simulink library "MATH_library"  (R2018b)
settings: Solver=VariableStepAuto  StartTime=0.0  StopTime=10.0  RelTol=1e-3
undefined symbols (not defined in the file): Newton, Raphson
libraries: $bdroot x48, sharedutil x4
(part 1 of 2)
settings Model: Creator=Andrea  LastModifiedBy=michele

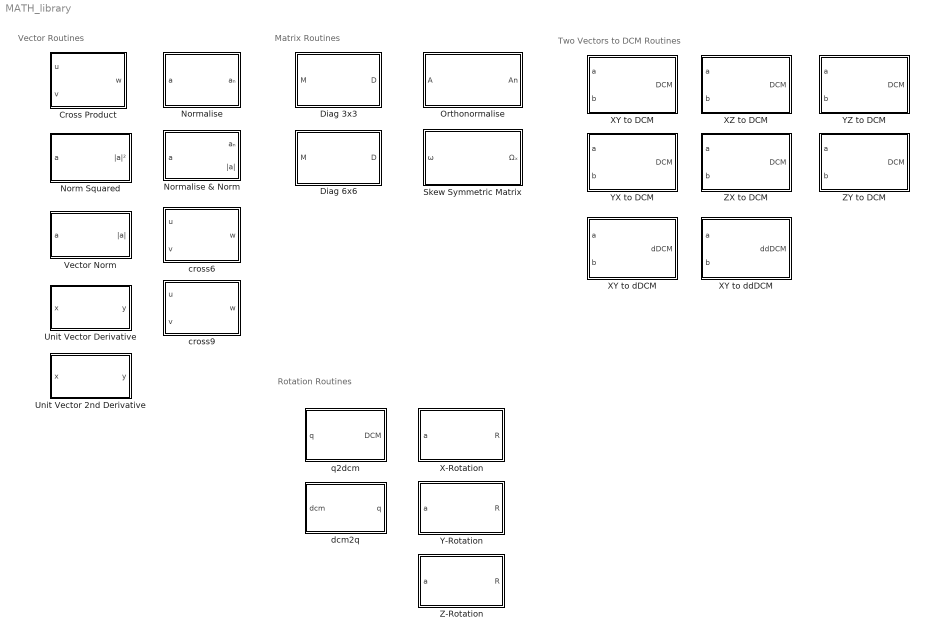
== system MATH_library ==
  note: Rotation Routines
  note: Matrix Routines
  note: Vector Routines
  note: Two Vectors to DCM Routines
  Cross Product : Subsystem  mask(Cross Product){}
      mask help: This block computes the cross product between two 3x1 input vectors u and v. The output vector w is such that w = u x v
  Diag 3x3 : Subsystem  mask(Diagonal - 3x3){}
      mask help: Extract the diagonal of a 3x3 matrix.
  Diag 6x6 : Subsystem  mask(Diagonal - 6x6){}
      mask help: Extract the diagonal of a 6x6 matrix.
  Norm Squared : Subsystem  mask(Norm Squared){}
      mask help: Compute the square of the norm of the input vector.
  Normalise : Subsystem  mask(Normalise){}
      mask help: Normalise the input vector.
  Normalise & Norm : Subsystem  mask(Normalise){}
      mask help: Normalise the input vector and also return its norm.
  Orthonormalise : Subsystem  mask(Matrix Orthonormalisation){}
      mask help: This block performs the Gram-Schmidt orthonormalisation process on the input matrix A. However, note that this block does not check whether the columns of A span a three-dimensional space.
  Skew Symmetric Matrix : Subsystem  mask(Skew Symmetric Matrix){}
      mask help: This block generates a skew-symmetric matrix W from the given input vector w. The output matrix is defined such that the cross product w x b can be written as W * b
  Unit Vector 2nd Derivative : Subsystem  mask(Unit vector derivative){}
      mask help: Compute the derivative of a unit vector.
  Unit Vector Derivative : Subsystem  mask(Unit vector derivative){}
      mask help: Compute the derivative of a unit vector.
  Vector Norm : Subsystem  mask(Vector Norm){}
      mask help: Compute the norm of the input vector.
  X-Rotation : Subsystem  mask(X - Rotation){}
      mask help: Compute the matrix for a PASSIVE rotation around the X-axis for a given angle [rad].
  XY to DCM : Subsystem  mask(XY to DCM){}
      mask help:
      | This block computes a DCM from a 3D right-handed orthogonal vector basis obtained from the input vector a and b.
      |
      | INPUTS:
      |   - Primary vector that will be aligned with the X-axis
      |   - Secondary vector. The component of this vector that is orthogonal to the primary vector will be aligned to the Y-axis.
      |
      | OUTPUTS:
      |  -  3x3 Rotation matrix from the axes in which a and b are defined to the new ones.
  XY to dDCM : Subsystem  mask(XY to dDCM){}
      mask help:
      | This block computes the derivative of a DCM from a 3D right-handed orthogonal vector basis obtained from the input vector a and b. These input vectors must be of 6-elements, with the last 3 the derivatives of the first three.
      |
      | INPUTS:
      |   - Primary vector that will be aligned with the X-axis.
      |   - Secondary vector. The component of this vector that is orthogonal to the primary vector will be aligned to the Y-axis.
      |
      | OUTPUTS:
      |  -  3x3 Rotation matrix from the axes in which a and b are defined to the new ones.
  XY to ddDCM : Subsystem  mask(XY to dDCM){}
      mask help:
      | This block computes the derivative of a DCM from a 3D right-handed orthogonal vector basis obtained from the input vector a and b. These input vectors must be of 6-elements, with the last 3 the derivatives of the first three.
      |
      | INPUTS:
      |   - Primary vector that will be aligned with the X-axis.
      |   - Secondary vector. The component of this vector that is orthogonal to the primary vector will be aligned to the Y-axis.
      |
      | OUTPUTS:
      |  -  3x3 Rotation matrix from the axes in which a and b are defined to the new ones.
  XZ to DCM : Subsystem  mask(XZ to DCM){}
      mask help:
      | This block computes a DCM from a 3D right-handed orthogonal vector basis obtained from the input vector a and b.
      |
      | INPUTS:
      |   - Primary vector that will be aligned with the X-axis
      |   - Secondary vector. The component of this vector that is orthogonal to the primary vector will be aligned to the Z-axis.
      |
      | OUTPUTS:
      |   -  3x3 Rotation matrix from the axes in which a and b are defined to the new ones.
  Y-Rotation : Subsystem  mask(Y - Rotation){}
      mask help: Compute the matrix for a PASSIVE rotation around the Y-axis for a given angle [rad].
  YX to DCM : Subsystem  mask(YX to DCM){}
      mask help:
      | This block computes a DCM from a 3D right-handed orthogonal vector basis obtained from the input vector a and b.
      |
      | INPUTS:
      |   - Primary vector that will be aligned with the Y-axis
      |   - Secondary vector. The component of this vector that is orthogonal to the primary vector will be aligned to the X-axis.
      |
      | OUTPUTS:
      |   -  3x3 Rotation matrix from the axes in which a and b are defined to the new ones.
  YZ to DCM : Subsystem  mask(YZ to DCM){}
      mask help:
      | This block computes a DCM from a 3D right-handed orthogonal vector basis obtained from the input vector a and b.
      |
      | INPUTS:
      |   - Primary vector that will be aligned with the Y-axis
      |   - Secondary vector. The component of this vector that is orthogonal to the primary vector will be aligned to the Z-axis.
      |
      | OUTPUTS:
      |   -  3x3 Rotation matrix from the axes in which a and b are defined to the new ones.
  Z-Rotation : Subsystem  mask(Z - Rotation){}
      mask help: Compute the matrix for a PASSIVE rotation around the Z-axis for a given angle [rad].
  ZX to DCM : Subsystem  mask(ZX to DCM){}
      mask help:
      | This block computes a DCM from a 3D right-handed orthogonal vector basis obtained from the input vector a and b.
      |
      | INPUTS:
      |   - Primary vector that will be aligned with the Z-axis
      |   - Secondary vector. The component of this vector that is orthogonal to the primary vector will be aligned to the X-axis.
      |
      | OUTPUTS:
      |   -  3x3 Rotation matrix from the axes in which a and b are defined to the new ones.
  ZY to DCM : Subsystem  mask(ZY to DCM){}
      mask help:
      | This block computes a DCM from a 3D right-handed orthogonal vector basis obtained from the input vector a and b.
      |
      | INPUTS:
      |   - Primary vector that will be aligned with the Z-axis
      |   - Secondary vector. The component of this vector that is orthogonal to the primary vector will be aligned to the Y-axis.
      |
      | OUTPUTS:
      |   -  3x3 Rotation matrix from the axes in which a and b are defined to the new ones.
  cross6 : Subsystem  mask(Cross 6){}
      mask help: Compute the cross product between two vectors and its time derivative. Each input vector must be of 6 elements, with the last 3 that represent the derivative of the first.
  cross9 : Subsystem  mask(Cross 6){}
      mask help: Compute the cross product between two vectors and its time derivative. Each input vector must be of 6 elements, with the last 3 that represent the derivative of the first.
  dcm2q : Subsystem  mask(DCM to Quaternion){}
      mask help: Convert a Direction Cosine Matrix (DCM) into a quaternion (in scalar-last format).
  q2dcm : Subsystem  mask(Quaternion to DCM){}
      mask help: Convert a quaternion (in scalar-last format) into a Direction Cosine Matrix (DCM)

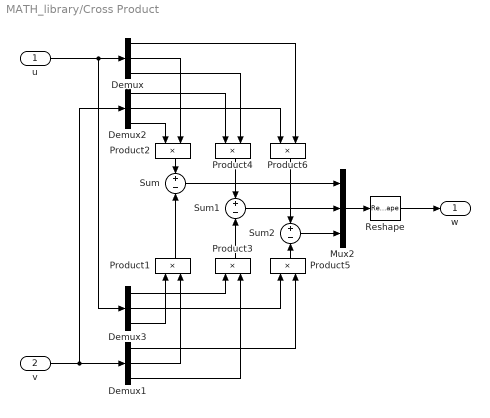
== system MATH_library/Cross Product ==
  u : Inport
  v : Inport  Port=2
  Demux{,1..3} (4 alike) : Demux  Outputs=3
  Mux2 : Mux  Inputs=3
  Product{1..6} (6 alike) : Product  SaturateOnIntegerOverflow=on  RndMeth=Zero  InputSameDT=on  OutDataTypeStr=Inherit: Same as first input
  Reshape : Reshape  OutputDimensionality=Column vector (2-D)
  Sum : Sum  Inputs=+-  SaturateOnIntegerOverflow=on  InputSameDT=on  OutDataTypeStr=Inherit: Same as first input
  Sum1 : Sum  Inputs=+-  SaturateOnIntegerOverflow=on  InputSameDT=on  OutDataTypeStr=Inherit: Same as first input
  Sum2 : Sum  Inputs=+-  SaturateOnIntegerOverflow=on  InputSameDT=on  OutDataTypeStr=Inherit: Same as first input
  w : Outport
  wires:
  Product6/1 -> Sum2/1
  Demux/2 -> Product2/2
  Demux2/1 -> Product4/1
  Product1/1 -> Sum/2
  Product4/1 -> Sum1/1
  Sum2/1 -> Mux2/3
  Sum1/1 -> Mux2/2
  Demux3/3 -> Product1/1
  u/1 -> Demux3/1, Demux/1
  Demux/3 -> Product4/2
  Product3/1 -> Sum1/2
  Mux2/1 -> Reshape/1
  Demux/1 -> Product6/2
  Demux1/2 -> Product1/2
  Product5/1 -> Sum2/2
  Sum/1 -> Mux2/1
  Demux1/1 -> Product5/2
  Product2/1 -> Sum/1
  Reshape/1 -> w/1
  v/1 -> Demux1/1, Demux2/1
  Demux2/2 -> Product6/1
  Demux1/3 -> Product3/2
  Demux3/2 -> Product5/1
  Demux3/1 -> Product3/1
  Demux2/3 -> Product2/1

== system MATH_library/Diag 3x3 ==
  M : Inport  OutDataTypeStr=single  PortDimensions=[3,3]
  Reshape : Reshape
  Selector : Selector  InputPortWidth=9  IndexOptions=Index vector (dialog)  Indices=[1 5 9]  OutputSizes=1
  D : Outport  OutDataTypeStr=single  PortDimensions=3
  wires:
  M/1 -> Reshape/1
  Reshape/1 -> Selector/1
  Selector/1 -> D/1

== system MATH_library/Diag 6x6 ==
  M : Inport  PortDimensions=[6,6]
  Reshape : Reshape
  Selector : Selector  InputPortWidth=36  IndexOptions=Index vector (dialog)  Indices=[1 8 15 22 29 36]  OutputSizes=1
  D : Outport  PortDimensions=6
  wires:
  M/1 -> Reshape/1
  Reshape/1 -> Selector/1
  Selector/1 -> D/1

== system MATH_library/Norm Squared ==
  a : Inport
  Dot Product : DotProduct  InputSameDT=on  OutDataTypeStr=Inherit: Inherit via internal rule
  |a|² : Outport
  wires:
  a/1 -> Dot Product/2, Dot Product/1
  Dot Product/1 -> |a|²/1

== system MATH_library/Normalise ==
  a : Inport
  Divide : Product  Inputs=*/
  Vector Norm : $bdroot/Vector Norm
  aₙ : Outport
  wires:
  a/1 -> Vector Norm/1, Divide/1
  Divide/1 -> aₙ/1
  Vector Norm/1 -> Divide/2

== system MATH_library/Normalise & Norm ==
  a : Inport
  Divide : Product  Inputs=*/
  Vector Norm : $bdroot/Vector Norm
  aₙ : Outport
  |a| : Outport  Port=2
  wires:
  a/1 -> Vector Norm/1, Divide/1
  Divide/1 -> aₙ/1
  Vector Norm/1 -> |a|/1, Divide/2

== system MATH_library/Orthonormalise ==
  A : Inport
  Demux : Demux  Outputs=3
  Normalise : $bdroot/Normalise
  Reshape : Reshape  OutputDimensionality=Column vector (2-D)
  Subsystem : Subsystem
  Subsystem1 : Subsystem
  Vector Concatenate : Concatenate  NumInputs=3  Mode=Multidimensional array  ConcatenateDimension=2
  An : Outport
  wires:
  A/1 -> Reshape/1
  Reshape/1 -> Demux/1
  Demux/1 -> Normalise/1  "e1"
  Normalise/1 -> Subsystem1/1(en1), Subsystem/1(en1), Vector Concatenate/1
  Demux/2 -> Subsystem/2(e2)  "e2"
  Demux/3 -> Subsystem1/2(e3)  "e3"
  Subsystem1/1(en3) -> Vector Concatenate/3
  Subsystem/1(en2) -> Subsystem1/3(en2), Vector Concatenate/2
  Vector Concatenate/1 -> An/1

== system MATH_library/Skew Symmetric Matrix ==
  ω : Inport
  Constant : Constant  Value=0
  Demux : Demux  Outputs=3
  Gain : Gain  Gain=-1
  Gain1 : Gain  Gain=-1
  Gain2 : Gain  Gain=-1
  Reshape (9) to [3x3] column-major : Reshape  OutputDimensionality=Customize  OutputDimensions=[3,3]
  Vector Concatenate : Concatenate  NumInputs=9
  Ωₓ : Outport
  wires:
  Constant/1 -> Vector Concatenate/9, Vector Concatenate/5, Vector Concatenate/1
  Demux/1 -> Vector Concatenate/6, Gain/1
  Reshape (9) to [3x3] column-major/1 -> Ωₓ/1
  Demux/3 -> Gain2/1, Vector Concatenate/2
  Demux/2 -> Vector Concatenate/7, Gain1/1
  ω/1 -> Demux/1
  Vector Concatenate/1 -> Reshape (9) to [3x3] column-major/1
  Gain1/1 -> Vector Concatenate/3
  Gain2/1 -> Vector Concatenate/4
  Gain/1 -> Vector Concatenate/8

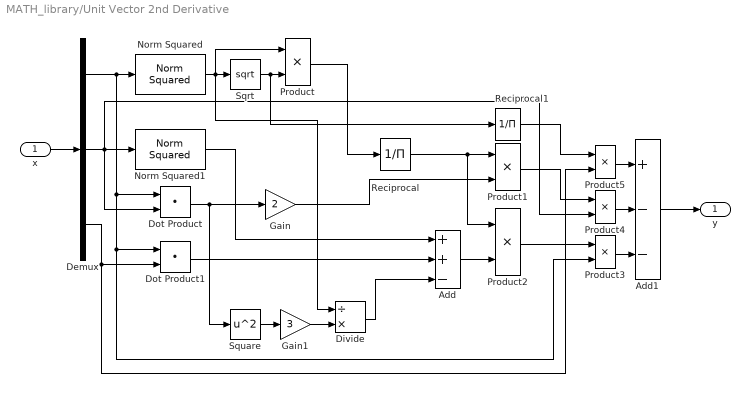
== system MATH_library/Unit Vector 2nd Derivative ==
  x : Inport
  Add : Sum  Inputs=++-
  Add1 : Sum  Inputs=+--
  Demux : Demux  Outputs=3
  Divide : Product  Inputs=/*
  Dot Product : DotProduct  InputSameDT=on  OutDataTypeStr=Inherit: Inherit via internal rule
  Dot Product1 : DotProduct  InputSameDT=on  OutDataTypeStr=Inherit: Inherit via internal rule
  Gain : Gain  Gain=2
  Gain1 : Gain  Gain=3
  Norm Squared : $bdroot/Norm Squared
  Norm Squared1 : $bdroot/Norm Squared
  Product{,1..5} (6 alike) : Product
  Reciprocal : Product  Inputs=/
  Reciprocal1 : Product  Inputs=/
  Sqrt : Sqrt  SaturateOnIntegerOverflow=on
  Square : Math  Operator=square  SaturateOnIntegerOverflow=on
  y : Outport
  wires:
  Add1/1 -> y/1
  x/1 -> Demux/1
  Demux/1 -> Norm Squared/1, Product3/2, Dot Product1/1, Dot Product/1
  Norm Squared/1 -> Divide/1, Product/1, Sqrt/1
  Sqrt/1 -> Reciprocal1/1, Product/2
  Demux/2 -> Product4/2, Dot Product/2, Norm Squared1/1
  Demux/3 -> Product5/2, Dot Product1/2
  Dot Product/1 -> Square/1, Gain/1
  Gain/1 -> Product1/2
  Reciprocal/1 -> Product2/1, Product1/1
  Product/1 -> Reciprocal/1
  Norm Squared1/1 -> Add/1
  Dot Product1/1 -> Add/2
  Square/1 -> Gain1/1
  Gain1/1 -> Divide/2
  Divide/1 -> Add/3
  Add/1 -> Product2/2
  Product2/1 -> Product3/1
  Product3/1 -> Add1/3
  Product4/1 -> Add1/2
  Product1/1 -> Product4/1
  Product5/1 -> Add1/1
  Reciprocal1/1 -> Product5/1

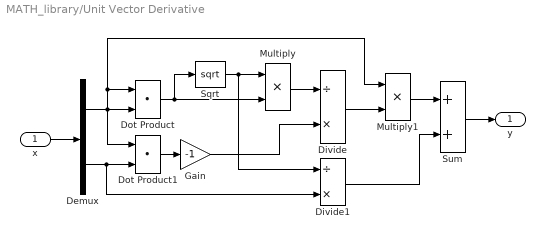
== system MATH_library/Unit Vector Derivative ==
  x : Inport
  Demux : Demux  Outputs=2
  Divide : Product  Inputs=/*
  Divide1 : Product  Inputs=/*
  Dot Product : DotProduct  InputSameDT=on  OutDataTypeStr=Inherit: Inherit via internal rule
  Dot Product1 : DotProduct  InputSameDT=on  OutDataTypeStr=Inherit: Inherit via internal rule
  Gain : Gain  Gain=-1
  Multiply : Product
  Multiply1 : Product
  Sqrt : Sqrt  SaturateOnIntegerOverflow=on
  Sum : Sum
  y : Outport
  wires:
  Divide/1 -> Multiply1/2
  Divide1/1 -> Sum/2
  Sum/1 -> y/1
  Multiply1/1 -> Sum/1
  Multiply/1 -> Divide/1
  Gain/1 -> Divide/2
  Demux/2 -> Divide1/2, Dot Product1/2
  Dot Product1/1 -> Gain/1
  Demux/1 -> Dot Product1/1, Multiply1/1, Dot Product/1, Dot Product/2
  Sqrt/1 -> Multiply/1, Divide1/1
  Dot Product/1 -> Multiply/2, Sqrt/1
  x/1 -> Demux/1

== system MATH_library/Vector Norm ==
  a : Inport
  Norm Squared : $bdroot/Norm Squared
  Sqrt : Sqrt  SaturateOnIntegerOverflow=on
  |a| : Outport
  wires:
  Sqrt/1 -> |a|/1
  Norm Squared/1 -> Sqrt/1
  a/1 -> Norm Squared/1

== system MATH_library/X-Rotation ==
  a : Inport
  Constant1 : Constant  Value=0
  Constant2 : Constant
  Constant3 : Constant  Value=0
  Constant4 : Constant
  Constant5 : Constant  Value=0
  Create 3x3 Matrix : sharedutil/Create 3x3 Matrix  aMode=aMode
  Gain : Gain  Gain=-1
  SinCos : Trigonometry  Operator=sincos
  R : Outport
  wires:
  a/1 -> SinCos/1
  Create 3x3 Matrix/1 -> R/1
  SinCos/2 -> Create 3x3 Matrix/9, Create 3x3 Matrix/5
  SinCos/1 -> Create 3x3 Matrix/6, Gain/1
  Constant3/1 -> Create 3x3 Matrix/2
  Constant4/1 -> Create 3x3 Matrix/1
  Constant5/1 -> Create 3x3 Matrix/3
  Constant2/1 -> Create 3x3 Matrix/7
  Constant1/1 -> Create 3x3 Matrix/4
  Gain/1 -> Create 3x3 Matrix/8

== system MATH_library/XY to DCM ==
  a : Inport
  b : Inport  Port=2
  " Matrix" : Concatenate  NumInputs=3  Mode=Multidimensional array  ConcatenateDimension=2
  Cross Product : $bdroot/Cross Product
  Cross Product1 : $bdroot/Cross Product
  Normalise : $bdroot/Normalise
  Normalise1 : $bdroot/Normalise
  Normalise2 : $bdroot/Normalise
  Transpose : Math  Operator=transpose  SaturateOnIntegerOverflow=on
  DCM : Outport
  wires:
  Normalise/1 -> " Matrix"/3  "w_n"
  Cross Product/1 -> Normalise/1, Cross Product1/1
  " Matrix"/1 -> Transpose/1
  Normalise2/1 -> " Matrix"/1  "u_n"
  Normalise1/1 -> " Matrix"/2  "v_n"
  b/1 -> Cross Product/2
  a/1 -> Normalise2/1, Cross Product/1, Cross Product1/2
  Cross Product1/1 -> Normalise1/1
  Transpose/1 -> DCM/1

== system MATH_library/XY to dDCM ==
  a : Inport
  b : Inport  Port=2
  " Matrix" : Concatenate  NumInputs=3  Mode=Multidimensional array  ConcatenateDimension=2
  Transpose : Math  Operator=transpose  SaturateOnIntegerOverflow=on
  Unit Vector Derivative : $bdroot/Unit Vector Derivative
  Unit Vector Derivative1 : $bdroot/Unit Vector Derivative
  Unit Vector Derivative2 : $bdroot/Unit Vector Derivative
  cross1 : $bdroot/cross6
  cross2 : $bdroot/cross6
  dDCM : Outport
  wires:
  Transpose/1 -> dDCM/1
  " Matrix"/1 -> Transpose/1
  cross2/1 -> Unit Vector Derivative1/1
  Unit Vector Derivative/1 -> " Matrix"/3
  cross1/1 -> Unit Vector Derivative/1, cross2/1
  b/1 -> cross1/2, cross2/2
  a/1 -> Unit Vector Derivative2/1, cross1/1
  Unit Vector Derivative2/1 -> " Matrix"/1
  Unit Vector Derivative1/1 -> " Matrix"/2

== system MATH_library/XY to ddDCM ==
  a : Inport
  b : Inport  Port=2
  " Matrix" : Concatenate  NumInputs=3  Mode=Multidimensional array  ConcatenateDimension=2
  Transpose : Math  Operator=transpose  SaturateOnIntegerOverflow=on
  Unit Vector 2nd Derivative : $bdroot/Unit Vector 2nd Derivative
  Unit Vector 2nd Derivative1 : $bdroot/Unit Vector 2nd Derivative
  Unit Vector 2nd Derivative2 : $bdroot/Unit Vector 2nd Derivative
  cross1 : $bdroot/cross9
  cross9 : $bdroot/cross9
  ddDCM : Outport
  wires:
  Transpose/1 -> ddDCM/1
  " Matrix"/1 -> Transpose/1
  cross1/1 -> Unit Vector 2nd Derivative1/1
  Unit Vector 2nd Derivative2/1 -> " Matrix"/3
  cross9/1 -> Unit Vector 2nd Derivative2/1, cross1/1
  b/1 -> cross1/2, cross9/2
  a/1 -> Unit Vector 2nd Derivative/1, cross9/1
  Unit Vector 2nd Derivative/1 -> " Matrix"/1
  Unit Vector 2nd Derivative1/1 -> " Matrix"/2

== system MATH_library/XZ to DCM ==
  a : Inport
  b : Inport  Port=2
  " Matrix" : Concatenate  NumInputs=3  Mode=Multidimensional array  ConcatenateDimension=2
  Cross Product1 : $bdroot/Cross Product
  Cross Product2 : $bdroot/Cross Product
  Normalise1 : $bdroot/Normalise
  Normalise2 : $bdroot/Normalise
  Normalise3 : $bdroot/Normalise
  Transpose : Math  Operator=transpose  SaturateOnIntegerOverflow=on
  DCM : Outport
  wires:
  Normalise1/1 -> " Matrix"/3  "w_n"
  " Matrix"/1 -> Transpose/1
  Normalise3/1 -> " Matrix"/1  "u_n"
  Normalise2/1 -> " Matrix"/2  "v_n"
  a/1 -> Normalise3/1, Cross Product2/2, Cross Product1/1
  Cross Product2/1 -> Cross Product1/2, Normalise2/1
  b/1 -> Cross Product2/1
  Cross Product1/1 -> Normalise1/1
  Transpose/1 -> DCM/1

== system MATH_library/Y-Rotation ==
  a : Inport
  Constant1 : Constant  Value=0
  Constant2 : Constant
  Constant3 : Constant  Value=0
  Constant4 : Constant
  Constant5 : Constant  Value=0
  Create 3x3 Matrix : sharedutil/Create 3x3 Matrix  aMode=aMode
  Gain : Gain  Gain=-1
  SinCos : Trigonometry  Operator=sincos
  R : Outport
  wires:
  a/1 -> SinCos/1
  Create 3x3 Matrix/1 -> R/1
  SinCos/2 -> Create 3x3 Matrix/9, Create 3x3 Matrix/1
  SinCos/1 -> Create 3x3 Matrix/7, Gain/1
  Gain/1 -> Create 3x3 Matrix/3
  Constant4/1 -> Create 3x3 Matrix/5
  Constant3/1 -> Create 3x3 Matrix/2
  Constant5/1 -> Create 3x3 Matrix/4
  Constant1/1 -> Create 3x3 Matrix/8
  Constant2/1 -> Create 3x3 Matrix/6

== system MATH_library/YX to DCM ==
  a : Inport
  b : Inport  Port=2
  " Matrix" : Concatenate  NumInputs=3  Mode=Multidimensional array  ConcatenateDimension=2
  Cross Product1 : $bdroot/Cross Product
  Cross Product2 : $bdroot/Cross Product
  Normalise1 : $bdroot/Normalise
  Normalise2 : $bdroot/Normalise
  Normalise3 : $bdroot/Normalise
  Transpose : Math  Operator=transpose  SaturateOnIntegerOverflow=on
  DCM : Outport
  wires:
  a/1 -> Cross Product1/2, Normalise2/1, Cross Product2/1
  Normalise2/1 -> " Matrix"/2  "v_n"
  Normalise3/1 -> " Matrix"/1  "u_n"
  " Matrix"/1 -> Transpose/1
  Cross Product1/1 -> Normalise1/1, Cross Product2/2
  Normalise1/1 -> " Matrix"/3  "w_n"
  b/1 -> Cross Product1/1
  Cross Product2/1 -> Normalise3/1
  Transpose/1 -> DCM/1

== system MATH_library/YZ to DCM ==
  a : Inport
  b : Inport  Port=2
  " Matrix" : Concatenate  NumInputs=3  Mode=Multidimensional array  ConcatenateDimension=2
  Cross Product1 : $bdroot/Cross Product
  Cross Product2 : $bdroot/Cross Product
  Normalise1 : $bdroot/Normalise
  Normalise2 : $bdroot/Normalise
  Normalise3 : $bdroot/Normalise
  Transpose : Math  Operator=transpose  SaturateOnIntegerOverflow=on
  DCM : Outport
  wires:
  Normalise2/1 -> " Matrix"/3  "w_n"
  " Matrix"/1 -> Transpose/1
  Normalise3/1 -> " Matrix"/1  "u_n"
  Normalise1/1 -> " Matrix"/2  "v_n"
  a/1 -> Cross Product1/2, Normalise1/1, Cross Product2/1
  Cross Product2/1 -> Normalise3/1, Cross Product1/1
  b/1 -> Cross Product2/2
  Cross Product1/1 -> Normalise2/1
  Transpose/1 -> DCM/1

== system MATH_library/Z-Rotation ==
  a : Inport
  Constant{1..3,5} (4 alike) : Constant  Value=0
  Constant4 : Constant
  Create 3x3 Matrix : sharedutil/Create 3x3 Matrix  aMode=aMode
  Gain : Gain  Gain=-1
  SinCos : Trigonometry  Operator=sincos
  R : Outport
  wires:
  a/1 -> SinCos/1
  Create 3x3 Matrix/1 -> R/1
  SinCos/2 -> Create 3x3 Matrix/5, Create 3x3 Matrix/1
  SinCos/1 -> Gain/1, Create 3x3 Matrix/2
  Constant5/1 -> Create 3x3 Matrix/3
  Constant1/1 -> Create 3x3 Matrix/8
  Constant2/1 -> Create 3x3 Matrix/7
  Constant3/1 -> Create 3x3 Matrix/6
  Constant4/1 -> Create 3x3 Matrix/9
  Gain/1 -> Create 3x3 Matrix/4

== system MATH_library/ZX to DCM ==
  a : Inport
  b : Inport  Port=2
  " Matrix" : Concatenate  NumInputs=3  Mode=Multidimensional array  ConcatenateDimension=2
  Cross Product1 : $bdroot/Cross Product
  Cross Product2 : $bdroot/Cross Product
  Normalise1 : $bdroot/Normalise
  Normalise2 : $bdroot/Normalise
  Normalise3 : $bdroot/Normalise
  Transpose : Math  Operator=transpose  SaturateOnIntegerOverflow=on
  DCM : Outport
  wires:
  Normalise1/1 -> " Matrix"/3  "w_n"
  " Matrix"/1 -> Transpose/1
  Normalise3/1 -> " Matrix"/1  "u_n"
  Normalise2/1 -> " Matrix"/2  "v_n"
  a/1 -> Normalise1/1, Cross Product2/2, Cross Product1/1
  Cross Product1/1 -> Normalise2/1, Cross Product2/1
  b/1 -> Cross Product1/2
  Cross Product2/1 -> Normalise3/1
  Transpose/1 -> DCM/1

== system MATH_library/ZY to DCM ==
  a : Inport
  b : Inport  Port=2
  " Matrix" : Concatenate  NumInputs=3  Mode=Multidimensional array  ConcatenateDimension=2
  Cross Product1 : $bdroot/Cross Product
  Cross Product2 : $bdroot/Cross Product
  Normalise1 : $bdroot/Normalise
  Normalise2 : $bdroot/Normalise
  Normalise3 : $bdroot/Normalise
  Transpose : Math  Operator=transpose  SaturateOnIntegerOverflow=on
  DCM : Outport
  wires:
  Normalise2/1 -> " Matrix"/3  "w_n"
  " Matrix"/1 -> Transpose/1
  Normalise3/1 -> " Matrix"/1  "u_n"
  Normalise1/1 -> " Matrix"/2  "v_n"
  a/1 -> Normalise2/1, Cross Product2/1, Cross Product1/2
  b/1 -> Cross Product1/1
  Cross Product2/1 -> Normalise1/1
  Cross Product1/1 -> Normalise3/1, Cross Product2/2
  Transpose/1 -> DCM/1

== system MATH_library/cross6 ==
  u : Inport
  v : Inport  Port=2
  Reshape : Reshape  OutputDimensionality=Column vector (2-D)
  Vector Concatenate : Concatenate  NumInputs=6
  w1 : Subsystem
  w2 : Subsystem
  w3 : Subsystem
  w4 : Subsystem
  w5 : Subsystem
  w6 : Subsystem
  w : Outport
  wires:
  w6/1(w6) -> Vector Concatenate/6
  w5/1(w5) -> Vector Concatenate/5
  w4/1(w4) -> Vector Concatenate/4
  w3/1(w3) -> Vector Concatenate/3
  w2/1(w2) -> Vector Concatenate/2
  w1/1(w1) -> Vector Concatenate/1
  Reshape/1 -> w/1
  Vector Concatenate/1 -> Reshape/1
  v/1 -> w6/2(v), w1/2(v), w2/2(v), w3/2(v), w4/2(v), w5/2(v)
  u/1 -> w3/1(u), w4/1(u), w5/1(u), w6/1(u), w2/1(u), w1/1(u)

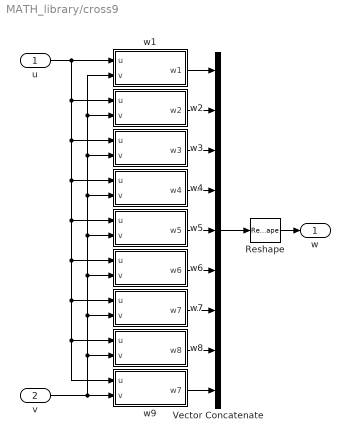
== system MATH_library/cross9 ==
  u : Inport
  v : Inport  Port=2
  Reshape : Reshape  OutputDimensionality=Column vector (2-D)
  Vector Concatenate : Concatenate  NumInputs=9
  w1 : Subsystem
  w2 : Subsystem
  w3 : Subsystem
  w4 : Subsystem
  w5 : Subsystem
  w6 : Subsystem
  w7 : Subsystem
  w8 : Subsystem
  w9 : Subsystem
  w : Outport
  wires:
  w6/1(w6) -> Vector Concatenate/6
  w5/1(w5) -> Vector Concatenate/5
  w4/1(w4) -> Vector Concatenate/4
  w3/1(w3) -> Vector Concatenate/3
  w2/1(w2) -> Vector Concatenate/2
  w1/1(w1) -> Vector Concatenate/1
  Reshape/1 -> w/1
  Vector Concatenate/1 -> Reshape/1
  v/1 -> w9/2(v), w8/2(v), w1/2(v), w2/2(v), w3/2(v), w4/2(v), w5/2(v), w6/2(v), w7/2(v)
  u/1 -> w3/1(u), w4/1(u), w5/1(u), w9/1(u), w8/1(u), w7/1(u), w6/1(u), w2/1(u), w1/1(u)
  w7/1(w7) -> Vector Concatenate/7
  w8/1(w8) -> Vector Concatenate/8
  w9/1(w7) -> Vector Concatenate/9

== system MATH_library/dcm2q ==
  dcm : Inport  Unit=1  PortDimensions=[3,3]
  If : If
  Merge : Merge  InitialOutput=[0; 0; 0; 1]
  Negative Trace : Subsystem
  Positive Trace : Subsystem
  "Reshape 3x3 -> 9" : Reshape  OutputDimensions=[9,1]
  trace : Subsystem
  q : Outport  Unit=1  PortDimensions=4
  wires:
  If/1 -> Positive Trace/Action
  Positive Trace/1(q) -> Merge/1
  Negative Trace/1(q) -> Merge/2
  If/2 -> Negative Trace/Action
  "Reshape 3x3 -> 9"/1 -> Negative Trace/1(DCM), Positive Trace/2(DCM), trace/1(DCM)
  dcm/1 -> "Reshape 3x3 -> 9"/1
  trace/1(trace(DCM)) -> Positive Trace/1(trace), If/1
  Merge/1 -> q/1

== system MATH_library/q2dcm ==
  q : Inport
  Create 3x3 Matrix : sharedutil/Create 3x3 Matrix  aMode=aMode
  Subsystem : Subsystem
  Subsystem1 : Subsystem
  Subsystem2 : Subsystem
  Subsystem3 : Subsystem
  Subsystem4 : Subsystem
  Subsystem5 : Subsystem
  Subsystem6 : Subsystem
  Subsystem7 : Subsystem
  Subsystem8 : Subsystem
  DCM : Outport
  wires:
  Subsystem3/1(A12) -> Create 3x3 Matrix/2
  Subsystem/1(A11) -> Create 3x3 Matrix/1
  Subsystem8/1(A23) -> Create 3x3 Matrix/6
  Subsystem2/1(A31) -> Create 3x3 Matrix/7
  Subsystem7/1(A32) -> Create 3x3 Matrix/8
  Subsystem1/1(A21) -> Create 3x3 Matrix/4
  Subsystem6/1(A13) -> Create 3x3 Matrix/3
  Subsystem4/1(A22) -> Create 3x3 Matrix/5
  Create 3x3 Matrix/1 -> DCM/1
  Subsystem5/1(A33) -> Create 3x3 Matrix/9
  q/1 -> Subsystem4/1(q), Subsystem1/1(q), Subsystem6/1(q), Subsystem3/1(q), Subsystem/1(q), Subsystem8/1(q), Subsystem2/1(q), Subsystem5/1(q), Subsystem7/1(q)

== system MATH_library/Orthonormalise/Subsystem ==
  en1 : Inport
  e2 : Inport  Port=2
  Dot Product : DotProduct  InputSameDT=on  OutDataTypeStr=Inherit: Inherit via internal rule
  Normalise : $bdroot/Normalise
  Product : Product
  Subtract : Sum  Inputs=-+
  en2 : Outport
  wires:
  Dot Product/1 -> Product/2
  Subtract/1 -> Normalise/1
  en1/1 -> Dot Product/1, Product/1
  e2/1 -> Dot Product/2, Subtract/2
  Product/1 -> Subtract/1
  Normalise/1 -> en2/1

== system MATH_library/Orthonormalise/Subsystem1 ==
  en1 : Inport
  e3 : Inport  Port=2
  en2 : Inport  Port=3
  Subsystem : Subsystem
  Subsystem1 : Subsystem
  en3 : Outport
  wires:
  e3/1 -> Subsystem/2(e3)
  Subsystem1/1(en3) -> en3/1
  en1/1 -> Subsystem/1(en1)
  en2/1 -> Subsystem1/1(en1)
  Subsystem/1(enj3) -> Subsystem1/2(enj3)

== system MATH_library/cross6/w1 ==
  note: u3*v2
  note: u2*v3
  u : Inport
  v : Inport  Port=2
  Demux : Demux  Outputs=2
  Demux1 : Demux  Outputs=2
  Multiply : Product
  Multiply1 : Product
  Selector : Selector  InputPortWidth=6  IndexOptions=Index vector (dialog)  Indices=[2 3]  OutputSizes=1
  Selector1 : Selector  InputPortWidth=6  IndexOptions=Index vector (dialog)  Indices=[2 3]  OutputSizes=1
  Subtract : Sum  Inputs=+-
  w1 : Outport
  wires:
  Demux/1 -> Multiply1/2
  Demux1/2 -> Multiply1/1
  Demux/2 -> Multiply/2
  Demux1/1 -> Multiply/1
  Selector/1 -> Demux1/1
  Selector1/1 -> Demux/1
  v/1 -> Selector1/1
  u/1 -> Selector/1
  Multiply1/1 -> Subtract/2
  Multiply/1 -> Subtract/1
  Subtract/1 -> w1/1

== system MATH_library/cross6/w2 ==
  note: u1*v3
  note: u3*v1
  u : Inport
  v : Inport  Port=2
  Demux : Demux  Outputs=2
  Demux1 : Demux  Outputs=2
  Multiply : Product
  Multiply1 : Product
  Selector : Selector  InputPortWidth=6  IndexOptions=Index vector (dialog)  Indices=[1 3]  OutputSizes=1
  Selector1 : Selector  InputPortWidth=6  IndexOptions=Index vector (dialog)  Indices=[1 3]  OutputSizes=1
  Subtract : Sum  Inputs=+-
  w2 : Outport
  wires:
  Demux/2 -> Multiply1/2
  Demux/1 -> Multiply/2
  Demux1/1 -> Multiply1/1
  Demux1/2 -> Multiply/1
  Selector/1 -> Demux1/1
  Selector1/1 -> Demux/1
  v/1 -> Selector1/1
  u/1 -> Selector/1
  Multiply1/1 -> Subtract/2
  Multiply/1 -> Subtract/1
  Subtract/1 -> w2/1

== system MATH_library/cross6/w3 ==
  note: u2*v1
  note: u1*v2
  u : Inport
  v : Inport  Port=2
  Demux : Demux  Outputs=2
  Demux1 : Demux  Outputs=2
  Multiply : Product
  Multiply1 : Product
  Selector : Selector  InputPortWidth=6  IndexOptions=Index vector (dialog)  Indices=[1 2]  OutputSizes=1
  Selector1 : Selector  InputPortWidth=6  IndexOptions=Index vector (dialog)  Indices=[1 2]  OutputSizes=1
  Subtract : Sum  Inputs=+-
  w3 : Outport
  wires:
  Demux/1 -> Multiply1/2
  Demux1/2 -> Multiply1/1
  Demux/2 -> Multiply/2
  Demux1/1 -> Multiply/1
  Selector/1 -> Demux1/1
  Selector1/1 -> Demux/1
  v/1 -> Selector1/1
  u/1 -> Selector/1
  Multiply1/1 -> Subtract/2
  Multiply/1 -> Subtract/1
  Subtract/1 -> w3/1

== system MATH_library/cross6/w4 ==
  note: u3*v5
  note: u6*v2
  note: u2*v6
  note: u5*v3
  u : Inport
  v : Inport  Port=2
  Demux1 : Demux
  Demux2 : Demux
  Multiply{,1..3} (4 alike) : Product
  Selector : Selector  InputPortWidth=6  IndexOptions=Index vector (dialog)  Indices=[2 3 5 6]  OutputSizes=1
  Selector1 : Selector  InputPortWidth=6  IndexOptions=Index vector (dialog)  Indices=[2 3 5 6]  OutputSizes=1
  Subtract : Sum  Inputs=++--
  w4 : Outport
  wires:
  Demux2/3 -> Multiply3/2
  Demux1/2 -> Multiply3/1
  Demux1/1 -> Multiply1/1
  Multiply3/1 -> Subtract/4
  Demux2/1 -> Multiply2/2
  Demux1/4 -> Multiply2/1
  Multiply2/1 -> Subtract/3
  Demux2/4 -> Multiply1/2
  Demux1/3 -> Multiply/1
  Demux2/2 -> Multiply/2
  Selector/1 -> Demux1/1
  Selector1/1 -> Demux2/1
  v/1 -> Selector1/1
  u/1 -> Selector/1
  Multiply1/1 -> Subtract/2
  Multiply/1 -> Subtract/1
  Subtract/1 -> w4/1

== system MATH_library/cross6/w5 ==
  note: u1*v6
  note: u4*v3
  note: u3*v4
  note: u6*v1
  u : Inport
  v : Inport  Port=2
  Demux1 : Demux
  Demux2 : Demux
  Multiply{,1..3} (4 alike) : Product
  Selector : Selector  InputPortWidth=6  IndexOptions=Index vector (dialog)  Indices=[1 3 4 6]  OutputSizes=1
  Selector1 : Selector  InputPortWidth=6  IndexOptions=Index vector (dialog)  Indices=[1 3 4 6]  OutputSizes=1
  Subtract : Sum  Inputs=++--
  w5 : Outport
  wires:
  Demux2/4 -> Multiply3/2
  Demux1/1 -> Multiply3/1
  Demux2/2 -> Multiply2/2
  Demux1/3 -> Multiply2/1
  Demux2/3 -> Multiply1/2
  Demux1/2 -> Multiply1/1
  Demux2/1 -> Multiply/2
  Demux1/4 -> Multiply/1
  Multiply3/1 -> Subtract/4
  Multiply2/1 -> Subtract/3
  Selector/1 -> Demux1/1
  Selector1/1 -> Demux2/1
  v/1 -> Selector1/1
  u/1 -> Selector/1
  Multiply1/1 -> Subtract/2
  Multiply/1 -> Subtract/1
  Subtract/1 -> w5/1

== system MATH_library/cross6/w6 ==
  note: u2*v4
  note: u5*v1
  note: u1*v5
  note: u4*v2
  u : Inport
  v : Inport  Port=2
  Demux1 : Demux
  Demux2 : Demux
  Multiply{,1..3} (4 alike) : Product
  Selector : Selector  InputPortWidth=6  IndexOptions=Index vector (dialog)  Indices=[1 2 4 5]  OutputSizes=1
  Selector1 : Selector  InputPortWidth=6  IndexOptions=Index vector (dialog)  Indices=[1 2 4 5]  OutputSizes=1
  Subtract : Sum  Inputs=++--
  w6 : Outport
  wires:
  Demux2/3 -> Multiply3/2
  Demux1/2 -> Multiply3/1
  Demux2/1 -> Multiply2/2
  Demux1/4 -> Multiply2/1
  Demux2/4 -> Multiply1/2
  Demux1/1 -> Multiply1/1
  Demux2/2 -> Multiply/2
  Demux1/3 -> Multiply/1
  Multiply3/1 -> Subtract/4
  Multiply2/1 -> Subtract/3
  Selector/1 -> Demux1/1
  Selector1/1 -> Demux2/1
  v/1 -> Selector1/1
  u/1 -> Selector/1
  Multiply1/1 -> Subtract/2
  Multiply/1 -> Subtract/1
  Subtract/1 -> w6/1

== system MATH_library/cross9/w1 ==
  note: u3*v2
  note: u2*v3
  u : Inport
  v : Inport  Port=2
  Demux : Demux  Outputs=2
  Demux1 : Demux  Outputs=2
  Multiply : Product
  Multiply1 : Product
  Selector : Selector  InputPortWidth=9  IndexOptions=Index vector (dialog)  Indices=[2 3]  OutputSizes=1
  Selector1 : Selector  InputPortWidth=9  IndexOptions=Index vector (dialog)  Indices=[2 3]  OutputSizes=1
  Subtract : Sum  Inputs=+-
  w1 : Outport
  wires:
  Demux/1 -> Multiply1/2
  Demux1/2 -> Multiply1/1
  Demux/2 -> Multiply/2
  Demux1/1 -> Multiply/1
  Selector/1 -> Demux1/1
  Selector1/1 -> Demux/1
  v/1 -> Selector1/1
  u/1 -> Selector/1
  Multiply1/1 -> Subtract/2
  Multiply/1 -> Subtract/1
  Subtract/1 -> w1/1

== system MATH_library/cross9/w2 ==
  note: u1*v3
  note: u3*v1
  u : Inport
  v : Inport  Port=2
  Demux : Demux  Outputs=2
  Demux1 : Demux  Outputs=2
  Multiply : Product
  Multiply1 : Product
  Selector : Selector  InputPortWidth=9  IndexOptions=Index vector (dialog)  Indices=[1 3]  OutputSizes=1
  Selector1 : Selector  InputPortWidth=9  IndexOptions=Index vector (dialog)  Indices=[1 3]  OutputSizes=1
  Subtract : Sum  Inputs=+-
  w2 : Outport
  wires:
  Demux/2 -> Multiply1/2
  Demux/1 -> Multiply/2
  Demux1/1 -> Multiply1/1
  Demux1/2 -> Multiply/1
  Selector/1 -> Demux1/1
  Selector1/1 -> Demux/1
  v/1 -> Selector1/1
  u/1 -> Selector/1
  Multiply1/1 -> Subtract/2
  Multiply/1 -> Subtract/1
  Subtract/1 -> w2/1

== system MATH_library/cross9/w3 ==
  note: u2*v1
  note: u1*v2
  u : Inport
  v : Inport  Port=2
  Demux : Demux  Outputs=2
  Demux1 : Demux  Outputs=2
  Multiply : Product
  Multiply1 : Product
  Selector : Selector  InputPortWidth=9  IndexOptions=Index vector (dialog)  Indices=[1 2]  OutputSizes=1
  Selector1 : Selector  InputPortWidth=9  IndexOptions=Index vector (dialog)  Indices=[1 2]  OutputSizes=1
  Subtract : Sum  Inputs=+-
  w3 : Outport
  wires:
  Demux/1 -> Multiply1/2
  Demux1/2 -> Multiply1/1
  Demux/2 -> Multiply/2
  Demux1/1 -> Multiply/1
  Selector/1 -> Demux1/1
  Selector1/1 -> Demux/1
  v/1 -> Selector1/1
  u/1 -> Selector/1
  Multiply1/1 -> Subtract/2
  Multiply/1 -> Subtract/1
  Subtract/1 -> w3/1

== system MATH_library/cross9/w4 ==
  note: u3*v5
  note: u6*v2
  note: u2*v6
  note: u5*v3
  u : Inport
  v : Inport  Port=2
  Demux1 : Demux
  Demux2 : Demux
  Multiply{,1..3} (4 alike) : Product
  Selector : Selector  InputPortWidth=9  IndexOptions=Index vector (dialog)  Indices=[2 3 5 6]  OutputSizes=1
  Selector1 : Selector  InputPortWidth=9  IndexOptions=Index vector (dialog)  Indices=[2 3 5 6]  OutputSizes=1
  Subtract : Sum  Inputs=++--
  w4 : Outport
  wires:
  Demux2/3 -> Multiply3/2
  Demux1/2 -> Multiply3/1
  Demux1/1 -> Multiply1/1
  Multiply3/1 -> Subtract/4
  Demux2/1 -> Multiply2/2
  Demux1/4 -> Multiply2/1
  Multiply2/1 -> Subtract/3
  Demux2/4 -> Multiply1/2
  Demux1/3 -> Multiply/1
  Demux2/2 -> Multiply/2
  Selector/1 -> Demux1/1
  Selector1/1 -> Demux2/1
  v/1 -> Selector1/1
  u/1 -> Selector/1
  Multiply1/1 -> Subtract/2
  Multiply/1 -> Subtract/1
  Subtract/1 -> w4/1

== system MATH_library/cross9/w5 ==
  note: u1*v6
  note: u4*v3
  note: u3*v4
  note: u6*v1
  u : Inport
  v : Inport  Port=2
  Demux1 : Demux
  Demux2 : Demux
  Multiply{,1..3} (4 alike) : Product
  Selector : Selector  InputPortWidth=9  IndexOptions=Index vector (dialog)  Indices=[1 3 4 6]  OutputSizes=1
  Selector1 : Selector  InputPortWidth=9  IndexOptions=Index vector (dialog)  Indices=[1 3 4 6]  OutputSizes=1
  Subtract : Sum  Inputs=++--
  w5 : Outport
  wires:
  Demux2/4 -> Multiply3/2
  Demux1/1 -> Multiply3/1
  Demux2/2 -> Multiply2/2
  Demux1/3 -> Multiply2/1
  Demux2/3 -> Multiply1/2
  Demux1/2 -> Multiply1/1
  Demux2/1 -> Multiply/2
  Demux1/4 -> Multiply/1
  Multiply3/1 -> Subtract/4
  Multiply2/1 -> Subtract/3
  Selector/1 -> Demux1/1
  Selector1/1 -> Demux2/1
  v/1 -> Selector1/1
  u/1 -> Selector/1
  Multiply1/1 -> Subtract/2
  Multiply/1 -> Subtract/1
  Subtract/1 -> w5/1

== system MATH_library/cross9/w6 ==
  note: u2*v4
  note: u5*v1
  note: u1*v5
  note: u4*v2
  u : Inport
  v : Inport  Port=2
  Demux1 : Demux
  Demux2 : Demux
  Multiply{,1..3} (4 alike) : Product
  Selector : Selector  InputPortWidth=9  IndexOptions=Index vector (dialog)  Indices=[1 2 4 5]  OutputSizes=1
  Selector1 : Selector  InputPortWidth=9  IndexOptions=Index vector (dialog)  Indices=[1 2 4 5]  OutputSizes=1
  Subtract : Sum  Inputs=++--
  w6 : Outport
  wires:
  Demux2/3 -> Multiply3/2
  Demux1/2 -> Multiply3/1
  Demux2/1 -> Multiply2/2
  Demux1/4 -> Multiply2/1
  Demux2/4 -> Multiply1/2
  Demux1/1 -> Multiply1/1
  Demux2/2 -> Multiply/2
  Demux1/3 -> Multiply/1
  Multiply3/1 -> Subtract/4
  Multiply2/1 -> Subtract/3
  Selector/1 -> Demux1/1
  Selector1/1 -> Demux2/1
  v/1 -> Selector1/1
  u/1 -> Selector/1
  Multiply1/1 -> Subtract/2
  Multiply/1 -> Subtract/1
  Subtract/1 -> w6/1

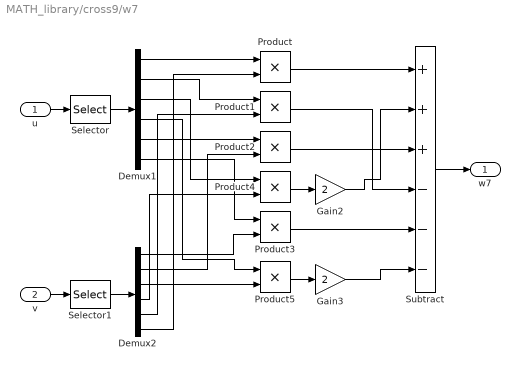
== system MATH_library/cross9/w7 ==
  u : Inport
  v : Inport  Port=2
  Demux1 : Demux  Outputs=6
  Demux2 : Demux  Outputs=6
  Gain2 : Gain  Gain=2
  Gain3 : Gain  Gain=2
  Product{,1..5} (6 alike) : Product
  Selector : Selector  InputPortWidth=9  IndexOptions=Index vector (dialog)  Indices=[2 3 5 6 8 9]  OutputSizes=1
  Selector1 : Selector  InputPortWidth=9  IndexOptions=Index vector (dialog)  Indices=[2 3 5 6 8 9]  OutputSizes=1
  Subtract : Sum  Inputs=+++---
  w7 : Outport
  wires:
  Selector/1 -> Demux1/1
  Selector1/1 -> Demux2/1
  v/1 -> Selector1/1
  u/1 -> Selector/1
  Subtract/1 -> w7/1
  Demux1/1 -> Product/1
  Demux2/6 -> Product/2
  Demux1/2 -> Product1/1
  Demux2/5 -> Product1/2
  Demux1/5 -> Product2/1
  Demux2/2 -> Product2/2
  Demux1/6 -> Product3/1
  Demux2/1 -> Product3/2
  Product4/1 -> Gain2/1
  Demux1/3 -> Product4/1
  Demux2/4 -> Product4/2
  Product5/1 -> Gain3/1
  Demux2/3 -> Product5/2
  Demux1/4 -> Product5/1
  Product/1 -> Subtract/1
  Product1/1 -> Subtract/4
  Product2/1 -> Subtract/3
  Product3/1 -> Subtract/5
  Gain3/1 -> Subtract/6
  Gain2/1 -> Subtract/2

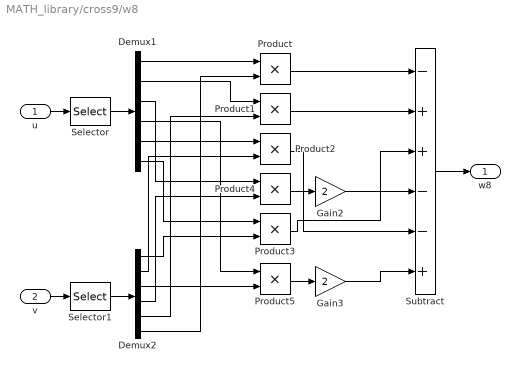
== system MATH_library/cross9/w8 ==
  u : Inport
  v : Inport  Port=2
  Demux1 : Demux  Outputs=6
  Demux2 : Demux  Outputs=6
  Gain2 : Gain  Gain=2
  Gain3 : Gain  Gain=2
  Product{,1..5} (6 alike) : Product
  Selector : Selector  InputPortWidth=9  IndexOptions=Index vector (dialog)  Indices=[1 3 4 6 7 9]  OutputSizes=1
  Selector1 : Selector  InputPortWidth=9  IndexOptions=Index vector (dialog)  Indices=[1 3 4 6 7 9]  OutputSizes=1
  Subtract : Sum  Inputs=-++--+
  w8 : Outport
  wires:
  Selector/1 -> Demux1/1
  Selector1/1 -> Demux2/1
  v/1 -> Selector1/1
  u/1 -> Selector/1
  Subtract/1 -> w8/1
  Product4/1 -> Gain2/1
  Demux1/1 -> Product/1
  Demux2/6 -> Product/2
  Product/1 -> Subtract/1
  Demux1/2 -> Product1/1
  Demux2/5 -> Product1/2
  Product1/1 -> Subtract/2
  Demux1/3 -> Product4/1
  Demux2/4 -> Product4/2
  Gain2/1 -> Subtract/4
  Demux1/4 -> Product5/1
  Demux2/3 -> Product5/2
  Product5/1 -> Gain3/1
  Gain3/1 -> Subtract/6
  Demux1/5 -> Product2/1
  Demux2/2 -> Product2/2
  Product2/1 -> Subtract/5
  Demux1/6 -> Product3/1
  Demux2/1 -> Product3/2
  Product3/1 -> Subtract/3

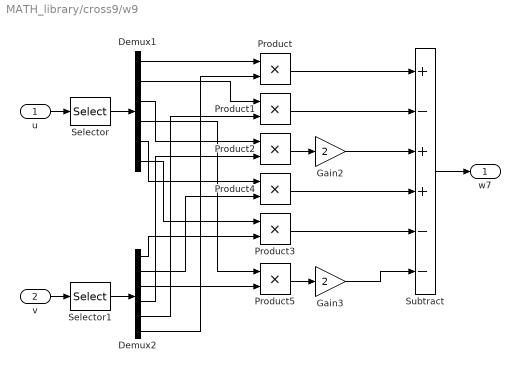
== system MATH_library/cross9/w9 ==
  u : Inport
  v : Inport  Port=2
  Demux1 : Demux  Outputs=6
  Demux2 : Demux  Outputs=6
  Gain2 : Gain  Gain=2
  Gain3 : Gain  Gain=2
  Product{,1..5} (6 alike) : Product
  Selector : Selector  InputPortWidth=9  IndexOptions=Index vector (dialog)  Indices=[1 2 4 5 7 8]  OutputSizes=1
  Selector1 : Selector  InputPortWidth=9  IndexOptions=Index vector (dialog)  Indices=[1 2 4 5 7 8]  OutputSizes=1
  Subtract : Sum  Inputs=+-++--
  w7 : Outport
  wires:
  Selector/1 -> Demux1/1
  Selector1/1 -> Demux2/1
  v/1 -> Selector1/1
  u/1 -> Selector/1
  Subtract/1 -> w7/1
  Demux1/1 -> Product/1
  Demux2/6 -> Product/2
  Product/1 -> Subtract/1
  Demux1/2 -> Product1/1
  Demux2/5 -> Product1/2
  Product1/1 -> Subtract/2
  Demux1/3 -> Product2/1
  Product2/1 -> Gain2/1
  Demux2/4 -> Product2/2
  Gain2/1 -> Subtract/3
  Demux1/4 -> Product5/1
  Demux2/3 -> Product5/2
  Product5/1 -> Gain3/1
  Gain3/1 -> Subtract/6
  Demux1/5 -> Product4/1
  Demux1/6 -> Product3/1
  Demux2/2 -> Product4/2
  Demux2/1 -> Product3/2
  Product3/1 -> Subtract/5
  Product4/1 -> Subtract/4

== system MATH_library/dcm2q/Negative Trace ==
  DCM : Inport
  Action Port : ActionPort  PropagateVarSize=During execution
  Demux : Demux  Outputs=3
  Find Maximum Diagonal Value : If  NumInputs=3  IfExpression=((u2 > u1) & (u2 > u3))  ElseIfExpressions=u3 > u1
  Maximum Value at DCM(1,1) : Subsystem
  Maximum Value at DCM(2,2) : Subsystem
  Maximum Value at DCM(3,3) : Subsystem
  Merge1 : Merge  Inputs=3  InitialOutput=[0; 0; 0; 1]
  Selector : Selector  InputPortWidth=9  IndexOptions=Index vector (dialog)  Indices=[1 5 9]  OutputSizes=1
  q : Outport
  wires:
  Maximum Value at DCM(1,1)/1(q) -> Merge1/3
  Merge1/1 -> q/1
  Find Maximum Diagonal Value/2 -> Maximum Value at DCM(3,3)/Action
  Maximum Value at DCM(2,2)/1(q) -> Merge1/1
  Find Maximum Diagonal Value/3 -> Maximum Value at DCM(1,1)/Action
  Demux/1 -> Find Maximum Diagonal Value/1
  Demux/3 -> Find Maximum Diagonal Value/3
  Maximum Value at DCM(3,3)/1(q) -> Merge1/2
  Demux/2 -> Find Maximum Diagonal Value/2
  DCM/1 -> Maximum Value at DCM(3,3)/1(DCM), Maximum Value at DCM(1,1)/1(DCM), Maximum Value at DCM(2,2)/1(DCM), Selector/1
  Find Maximum Diagonal Value/1 -> Maximum Value at DCM(2,2)/Action
  Selector/1 -> Demux/1

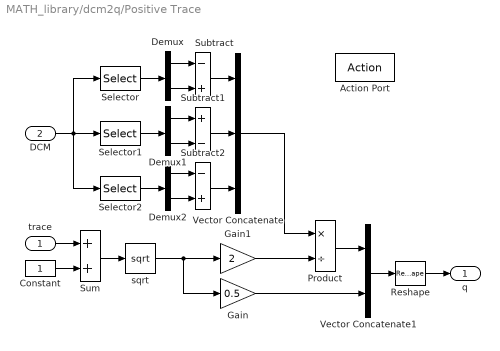
== system MATH_library/dcm2q/Positive Trace ==
  trace : Inport
  DCM : Inport  Port=2
  Action Port : ActionPort  PropagateVarSize=During execution
  Constant : Constant  OutDataTypeStr=Inherit: Inherit via back propagation
  Demux : Demux  Outputs=2
  Demux1 : Demux  Outputs=2
  Demux2 : Demux  Outputs=2
  Gain : Gain  Gain=0.5  OutDataTypeStr=Inherit: Inherit via back propagation  SaturateOnIntegerOverflow=on  ParamDataTypeStr=Inherit: Same as input
  Gain1 : Gain  Gain=2  OutDataTypeStr=Inherit: Inherit via back propagation  SaturateOnIntegerOverflow=on  ParamDataTypeStr=Inherit: Same as input
  Product : Product  Inputs=*/  SaturateOnIntegerOverflow=on  InputSameDT=on  OutDataTypeStr=Inherit: Same as first input
  Reshape : Reshape  OutputDimensionality=Column vector (2-D)
  Selector : Selector  InputPortWidth=9  IndexOptions=Index vector (dialog)  Indices=[6 8]  OutputSizes=1
  Selector1 : Selector  InputPortWidth=9  IndexOptions=Index vector (dialog)  Indices=[3 7]  OutputSizes=1
  Selector2 : Selector  InputPortWidth=9  IndexOptions=Index vector (dialog)  Indices=[2 4]  OutputSizes=1
  Subtract : Sum  Inputs=-+
  Subtract1 : Sum  Inputs=+-
  Subtract2 : Sum  Inputs=-+
  Sum : Sum  SaturateOnIntegerOverflow=on  InputSameDT=on  OutDataTypeStr=Inherit: Same as first input
  Vector Concatenate : Concatenate  NumInputs=3
  Vector Concatenate1 : Concatenate
  sqrt : Sqrt  AlgorithmType=Newton-Raphson  SaturateOnIntegerOverflow=on
  q : Outport
  wires:
  Constant/1 -> Sum/2
  Vector Concatenate/1 -> Product/1
  Gain1/1 -> Product/2
  trace/1 -> Sum/1
  Subtract2/1 -> Vector Concatenate/3
  Sum/1 -> sqrt/1
  DCM/1 -> Selector2/1, Selector1/1, Selector/1
  Subtract/1 -> Vector Concatenate/1
  sqrt/1 -> Gain/1, Gain1/1
  Subtract1/1 -> Vector Concatenate/2
  Product/1 -> Vector Concatenate1/1
  Gain/1 -> Vector Concatenate1/2
  Vector Concatenate1/1 -> Reshape/1
  Demux/1 -> Subtract/1
  Selector/1 -> Demux/1
  Demux/2 -> Subtract/2
  Demux1/2 -> Subtract1/2
  Selector1/1 -> Demux1/1
  Demux1/1 -> Subtract1/1
  Demux2/2 -> Subtract2/2
  Selector2/1 -> Demux2/1
  Demux2/1 -> Subtract2/1
  Reshape/1 -> q/1

== system MATH_library/dcm2q/trace ==
  DCM : Inport
  Selector : Selector  InputPortWidth=9  IndexOptions=Index vector (dialog)  Indices=[1 5 9]  OutputSizes=1
  Sum of Elements : Sum  Inputs=+
  trace(DCM) : Outport
  wires:
  Sum of Elements/1 -> trace(DCM)/1
  DCM/1 -> Selector/1
  Selector/1 -> Sum of Elements/1

== system MATH_library/q2dcm/Subsystem ==
  q : Inport
  Constant : Constant
  Gain : Gain  Gain=2
  Selector : Selector  InputPortWidth=4  IndexOptions=Index vector (dialog)  Indices=[2 3]  OutputSizes=1
  Square : Math  Operator=square  SaturateOnIntegerOverflow=on
  Sum : Sum  Inputs=+-
  Sum of Elements : Sum  Inputs=+
  A11 : Outport
  wires:
  Selector/1 -> Square/1
  Sum of Elements/1 -> Gain/1
  Sum/1 -> A11/1
  q/1 -> Selector/1
  Gain/1 -> Sum/2
  Square/1 -> Sum of Elements/1
  Constant/1 -> Sum/1

== system MATH_library/q2dcm/Subsystem1 ==
  q : Inport
  Add : Sum  Inputs=+-
  Demux : Demux
  Gain : Gain  Gain=2
  Multiply : Product
  Multiply1 : Product
  A21 : Outport
  wires:
  Gain/1 -> A21/1
  q/1 -> Demux/1
  Demux/1 -> Multiply/1
  Demux/2 -> Multiply/2
  Demux/3 -> Multiply1/1
  Demux/4 -> Multiply1/2
  Multiply/1 -> Add/1
  Multiply1/1 -> Add/2
  Add/1 -> Gain/1

== system MATH_library/q2dcm/Subsystem2 ==
  q : Inport
  Add : Sum
  Demux : Demux
  Gain : Gain  Gain=2
  Multiply : Product
  Multiply1 : Product
  A31 : Outport
  wires:
  Gain/1 -> A31/1
  q/1 -> Demux/1
  Multiply/1 -> Add/1
  Multiply1/1 -> Add/2
  Add/1 -> Gain/1
  Demux/1 -> Multiply/1
  Demux/3 -> Multiply/2
  Demux/2 -> Multiply1/1
  Demux/4 -> Multiply1/2

== system MATH_library/q2dcm/Subsystem3 ==
  q : Inport
  Add : Sum
  Demux : Demux
  Gain : Gain  Gain=2
  Multiply : Product
  Multiply1 : Product
  A12 : Outport
  wires:
  Gain/1 -> A12/1
  q/1 -> Demux/1
  Demux/1 -> Multiply/1
  Demux/2 -> Multiply/2
  Demux/3 -> Multiply1/1
  Demux/4 -> Multiply1/2
  Multiply/1 -> Add/1
  Multiply1/1 -> Add/2
  Add/1 -> Gain/1

== system MATH_library/q2dcm/Subsystem4 ==
  q : Inport
  Constant : Constant
  Gain : Gain  Gain=2
  Selector : Selector  InputPortWidth=4  IndexOptions=Index vector (dialog)  Indices=[1 3]  OutputSizes=1
  Square : Math  Operator=square  SaturateOnIntegerOverflow=on
  Sum : Sum  Inputs=+-
  Sum of Elements : Sum  Inputs=+
  A22 : Outport
  wires:
  Selector/1 -> Square/1
  Sum of Elements/1 -> Gain/1
  Sum/1 -> A22/1
  q/1 -> Selector/1
  Gain/1 -> Sum/2
  Square/1 -> Sum of Elements/1
  Constant/1 -> Sum/1

== system MATH_library/q2dcm/Subsystem5 ==
  q : Inport
  Constant : Constant
  Gain : Gain  Gain=2
  Selector : Selector  InputPortWidth=4  IndexOptions=Index vector (dialog)  Indices=[1 2]  OutputSizes=1
  Square : Math  Operator=square  SaturateOnIntegerOverflow=on
  Sum : Sum  Inputs=+-
  Sum of Elements : Sum  Inputs=+
  A33 : Outport
  wires:
  Selector/1 -> Square/1
  Sum of Elements/1 -> Gain/1
  Sum/1 -> A33/1
  q/1 -> Selector/1
  Gain/1 -> Sum/2
  Square/1 -> Sum of Elements/1
  Constant/1 -> Sum/1

== system MATH_library/q2dcm/Subsystem6 ==
  q : Inport
  Add : Sum  Inputs=+-
  Demux : Demux
  Gain : Gain  Gain=2
  Multiply : Product
  Multiply1 : Product
  A13 : Outport
  wires:
  Gain/1 -> A13/1
  q/1 -> Demux/1
  Multiply/1 -> Add/1
  Multiply1/1 -> Add/2
  Add/1 -> Gain/1
  Demux/1 -> Multiply/1
  Demux/3 -> Multiply/2
  Demux/2 -> Multiply1/1
  Demux/4 -> Multiply1/2

== system MATH_library/q2dcm/Subsystem7 ==
  q : Inport
  Add : Sum  Inputs=-+
  Demux : Demux
  Gain : Gain  Gain=2
  Multiply : Product
  Multiply1 : Product
  A32 : Outport
  wires:
  Gain/1 -> A32/1
  q/1 -> Demux/1
  Multiply/1 -> Add/1
  Multiply1/1 -> Add/2
  Add/1 -> Gain/1
  Demux/1 -> Multiply/1
  Demux/2 -> Multiply1/1
  Demux/3 -> Multiply1/2
  Demux/4 -> Multiply/2

== system MATH_library/q2dcm/Subsystem8 ==
  q : Inport
  Add : Sum
  Demux : Demux
  Gain : Gain  Gain=2
  Multiply : Product
  Multiply1 : Product
  A23 : Outport
  wires:
  Gain/1 -> A23/1
  q/1 -> Demux/1
  Multiply/1 -> Add/1
  Multiply1/1 -> Add/2
  Add/1 -> Gain/1
  Demux/1 -> Multiply/1
  Demux/2 -> Multiply1/1
  Demux/3 -> Multiply1/2
  Demux/4 -> Multiply/2

== system MATH_library/Orthonormalise/Subsystem1/Subsystem ==
  en1 : Inport
  e3 : Inport  Port=2
  Dot Product : DotProduct  InputSameDT=on  OutDataTypeStr=Inherit: Inherit via internal rule
  Product : Product
  Subtract : Sum  Inputs=-+
  enj3 : Outport
  wires:
  Dot Product/1 -> Product/2
  en1/1 -> Dot Product/1, Product/1
  e3/1 -> Dot Product/2, Subtract/2
  Product/1 -> Subtract/1
  Subtract/1 -> enj3/1

== system MATH_library/Orthonormalise/Subsystem1/Subsystem1 ==
  en1 : Inport
  enj3 : Inport  Port=2
  Dot Product : DotProduct  InputSameDT=on  OutDataTypeStr=Inherit: Inherit via internal rule
  Normalise : $bdroot/Normalise
  Product : Product
  Subtract : Sum  Inputs=-+
  en3 : Outport
  wires:
  Dot Product/1 -> Product/2
  Subtract/1 -> Normalise/1
  en1/1 -> Dot Product/1, Product/1
  enj3/1 -> Dot Product/2, Subtract/2
  Product/1 -> Subtract/1
  Normalise/1 -> en3/1

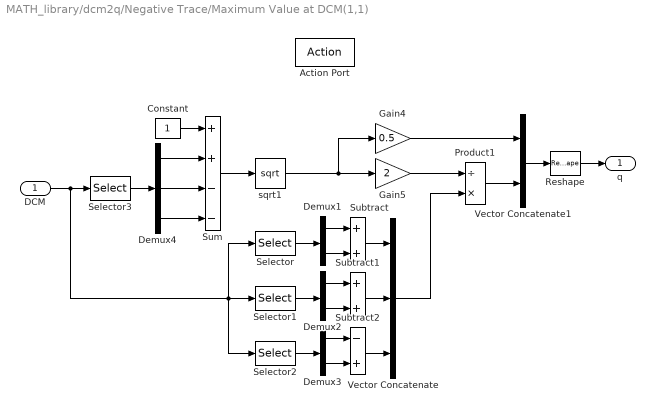
== system MATH_library/dcm2q/Negative Trace/Maximum Value at DCM(1,1) ==
  DCM : Inport
  Action Port : ActionPort  PropagateVarSize=During execution
  Constant : Constant
  Demux1 : Demux  Outputs=2
  Demux2 : Demux  Outputs=2
  Demux3 : Demux  Outputs=2
  Demux4 : Demux  Outputs=3
  Gain4 : Gain  Gain=0.5  OutDataTypeStr=Inherit: Inherit via back propagation  SaturateOnIntegerOverflow=on  ParamDataTypeStr=Inherit: Same as input
  Gain5 : Gain  Gain=2  OutDataTypeStr=Inherit: Inherit via back propagation  SaturateOnIntegerOverflow=on  ParamDataTypeStr=Inherit: Same as input
  Product1 : Product  Inputs=/*  SaturateOnIntegerOverflow=on  InputSameDT=on  OutDataTypeStr=Inherit: Same as first input
  Reshape : Reshape  OutputDimensionality=Column vector (2-D)
  Selector : Selector  InputPortWidth=9  IndexOptions=Index vector (dialog)  Indices=[2 4]  OutputSizes=1
  Selector1 : Selector  InputPortWidth=9  IndexOptions=Index vector (dialog)  Indices=[3 7]  OutputSizes=1
  Selector2 : Selector  InputPortWidth=9  IndexOptions=Index vector (dialog)  Indices=[6 8]  OutputSizes=1
  Selector3 : Selector  InputPortWidth=9  IndexOptions=Index vector (dialog)  Indices=[1 5 9]  OutputSizes=1
  Subtract : Sum
  Subtract1 : Sum
  Subtract2 : Sum  Inputs=-+
  Sum : Sum  Inputs=++--  SaturateOnIntegerOverflow=on  InputSameDT=on  OutDataTypeStr=Inherit: Same as first input
  Vector Concatenate : Concatenate  NumInputs=3
  Vector Concatenate1 : Concatenate
  sqrt1 : Sqrt  AlgorithmType=Newton-Raphson  SaturateOnIntegerOverflow=on
  q : Outport
  wires:
  Vector Concatenate1/1 -> Reshape/1
  Subtract2/1 -> Vector Concatenate/3
  Demux2/2 -> Subtract1/2
  Demux2/1 -> Subtract1/1
  sqrt1/1 -> Gain4/1, Gain5/1
  Demux3/1 -> Subtract2/1
  Subtract1/1 -> Vector Concatenate/2
  Selector/1 -> Demux1/1
  Demux3/2 -> Subtract2/2
  Subtract/1 -> Vector Concatenate/1
  Demux1/2 -> Subtract/2
  Sum/1 -> sqrt1/1
  Demux1/1 -> Subtract/1
  Selector1/1 -> Demux2/1
  Selector2/1 -> Demux3/1
  DCM/1 -> Selector/1, Selector2/1, Selector1/1, Selector3/1
  Reshape/1 -> q/1
  Gain4/1 -> Vector Concatenate1/1
  Gain5/1 -> Product1/1
  Product1/1 -> Vector Concatenate1/2
  Vector Concatenate/1 -> Product1/2
  Selector3/1 -> Demux4/1
  Demux4/3 -> Sum/4
  Demux4/2 -> Sum/3
  Demux4/1 -> Sum/2
  Constant/1 -> Sum/1
